simulink model "definitivo"  (R2023a)
settings: Solver=VariableStepAuto  StartTime=0.0  StopTime=T_sim  RelTol=1e-3
values from neighbouring files (symbols this model uses):
  k = 1    [main.m]
  mu = 0.5    [main.m]
undefined symbols (not defined in the file or in its folder): A_tubo, base_barile, c, d_tubo, do_percent, g, gamma_l, h_limite, k_imbocco, k_uscita, kg_to_m, l, L_tubo, livello_0, m_to_kg, mu_l, p1, p2, r, r_grande, r_piccolo, rho_l, step_liq, step_time, theta_grande, theta_piccolo, up_percent, z1, z2
libraries: simulink x8
settings Model: Creator=PaoloA  LastModifiedBy=PaoloA

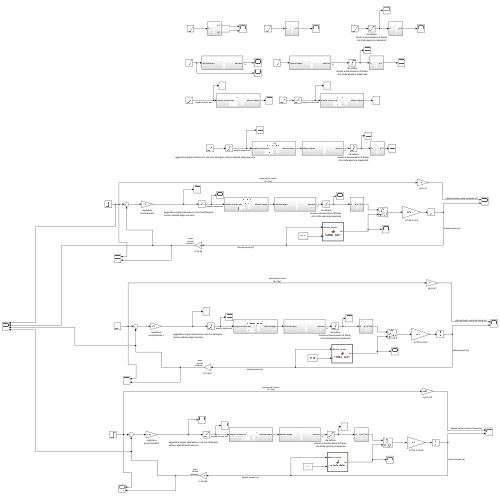
[thumbnail: Simulink's stored preview of the top-level diagram]
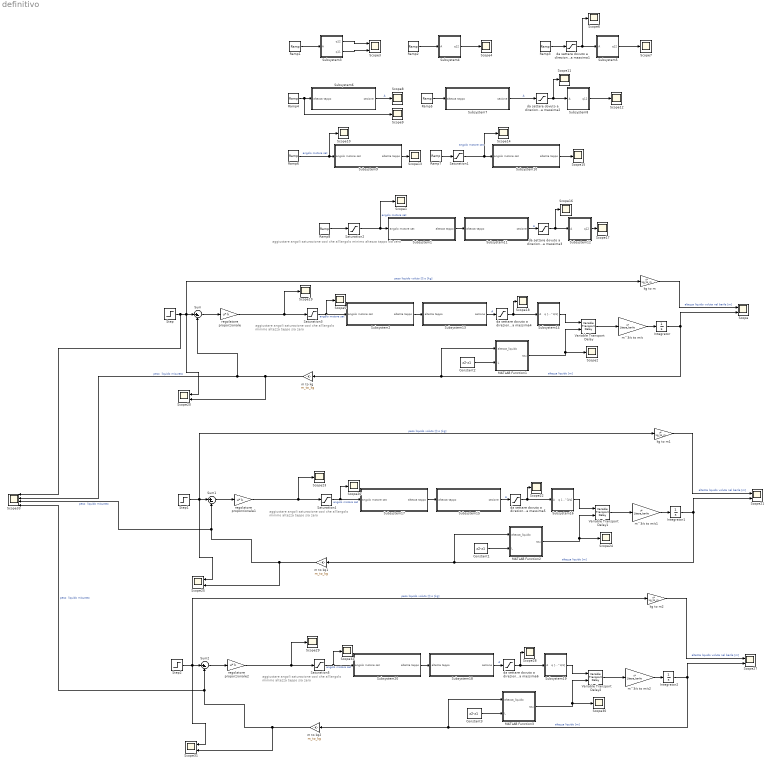
== system definitivo ==
  note: aggiustare angoli saturazione così che all'angolo minimo altezza tappo sia zero
  note: aggiustare angoli saturazione così che all'angolo
      | minimo altezza tappo sia zero
  note: aggiustare angoli saturazione così che all'angolo
      | minimo altezza tappo sia zero
  note: aggiustare angoli saturazione così che all'angolo
      | minimo altezza tappo sia zero
  Constant1 : Constant  Value=z2-z1
  Constant2 : Constant  Value=z2-z1
  Constant3 : Constant  Value=z2-z1
  Integrator : Integrator  InitialCondition=livello_0
  Integrator1 : Integrator  InitialCondition=livello_0
  Integrator2 : Integrator  InitialCondition=livello_0
  MATLAB Function1 : MATLAB Function  TreatAsAtomicUnit=on
  MATLAB Function2 : MATLAB Function  TreatAsAtomicUnit=on
  MATLAB Function3 : MATLAB Function  TreatAsAtomicUnit=on
  Ramp1 : simulink/Sources/Ramp  slope=0.00001  start=5  InitialOutput=0
  Ramp2 : simulink/Sources/Ramp  slope=0.00001  start=5  InitialOutput=0
  Ramp3 : simulink/Sources/Ramp  slope=0.00001  start=5  InitialOutput=0
  Ramp4 : simulink/Sources/Ramp  slope=0.0005  start=5  InitialOutput=0
  Ramp5 : simulink/Sources/Ramp  slope=0.0005  start=5  InitialOutput=0
  Ramp6 : simulink/Sources/Ramp  slope=0.2  start=5  InitialOutput=0
  Ramp7 : simulink/Sources/Ramp  slope=0.03  start=5  InitialOutput=0
  Ramp8 : simulink/Sources/Ramp  slope=0.03  start=5  InitialOutput=0
  Saturation{1..5} (5 alike) : Saturate  UpperLimit=pi  LowerLimit=0.01
  Scope{,3,20..21,25,27,31} (7 alike) : Scope  NumInputPorts=2
  Scope{1..2,4..19,22..24,26,28..30,32} (26 alike) : Scope
  Scope33 : Scope  NumInputPorts=4
  Step : Step  Time=step_time  After=step_liq  SampleTime=0
  Step1 : Step  Time=step_time  After=step_liq  SampleTime=0
  Step2 : Step  Time=step_time  After=step_liq  SampleTime=0
  Subsystem1 : Subsystem
  Subsystem10 : Subsystem
  Subsystem11 : Subsystem
  Subsystem12 : Subsystem
  Subsystem13 : Subsystem
  Subsystem14 : Subsystem
  Subsystem15 : Subsystem
  Subsystem16 : Subsystem
  Subsystem17 : Subsystem
  Subsystem18 : Subsystem
  Subsystem19 : Subsystem
  Subsystem2 : Subsystem
  Subsystem20 : Subsystem
  Subsystem3 : Subsystem
  Subsystem4 : Subsystem
  Subsystem5 : Subsystem
  Subsystem6 : Subsystem
  Subsystem7 : Subsystem
  Subsystem8 : Subsystem
  Subsystem9 : Subsystem
  Sum : Sum  Inputs=|+-
  Sum1 : Sum  Inputs=|+-
  Sum2 : Sum  Inputs=|+-
  Variable Transport Delay : VariableTransportDelay  MaximumDelay=tau_max
  Variable Transport Delay1 : VariableTransportDelay  MaximumDelay=tau_max
  Variable Transport Delay2 : VariableTransportDelay  MaximumDelay=tau_max
  da settare dovuto a direzionatore di flusso che limita apertura massima{1..6} (6 alike) : Saturate  UpperLimit=100  LowerLimit=0
  kg to m : Gain  Gain=kg_to_m  Multiplication=Matrix(u*K)
  kg to m1 : Gain  Gain=kg_to_m  Multiplication=Matrix(u*K)
  kg to m2 : Gain  Gain=kg_to_m  Multiplication=Matrix(u*K)
  m to kg : Gain  Gain=m_to_kg
  m to kg1 : Gain  Gain=m_to_kg
  m to kg2 : Gain  Gain=m_to_kg
  m^3/s to m/s : Gain  Gain=1/base_barile  Multiplication=Matrix(u*K)
  m^3/s to m/s1 : Gain  Gain=1/base_barile  Multiplication=Matrix(u*K)
  m^3/s to m/s2 : Gain  Gain=1/base_barile  Multiplication=Matrix(u*K)
  regolatore proporzionale : Gain  Gain=k  Multiplication=Matrix(u*K)
  regolatore proporzionale1 : Gain  Gain=k  Multiplication=Matrix(u*K)
  regolatore proporzionale2 : Gain  Gain=k  Multiplication=Matrix(u*K)
  wires:
  Subsystem3/1(q12) -> Scope3/1
  Subsystem4/1(q12) -> Scope4/1
  Sum/1 -> regolatore proporzionale/1
  Subsystem11/1(sezione) -> da settare dovuto a direzionatore di flusso che limita apertura massima3/1  "A"
  Step/1 -> Scope33/1, Scope20/1, kg to m/1, Sum/1  "peso liquido voluto [l] o [kg]"
  Ramp6/1 -> Scope10/1, Subsystem9/1(angolo motore sat)  "angolo motore sat"
  Subsystem12/1(q12) -> Scope17/1
  Integrator/1 -> m to kg/1, MATLAB Function1/1(altezza_liquido), Scope/2  "altezza liquido [m]"
  Subsystem9/1(altezza tappo) -> Scope13/1
  Saturation3/1 -> Subsystem2/1(angolo motore sat), Scope5/1  "angolo motore sat"
  regolatore proporzionale/1 -> Scope19/1, Saturation3/1
  Subsystem2/1(altezza tappo) -> Subsystem13/1(altezza tappo)
  MATLAB Function1/1(tau) -> Variable Transport Delay/2, Scope2/1
  da settare dovuto a direzionatore di flusso che limita apertura massima4/1 -> Scope18/1, Subsystem14/1(A)
  m to kg/1 -> Scope33/2, Sum/2, Scope20/2  "peso  liquido misurato"
  m^3/s to m/s/1 -> Integrator/1
  Ramp2/1 -> Subsystem4/1(A)
  Constant2/1 -> MATLAB Function1/2(L)
  Ramp7/1 -> Saturation1/1
  Subsystem8/1(q12) -> Scope12/1
  Saturation2/1 -> Scope1/1, Subsystem1/1(angolo motore sat)  "angolo motore sat"
  Subsystem1/1(altezza tappo) -> Subsystem11/1(altezza tappo)
  Ramp5/1 -> Subsystem7/1(altezza tappo)
  Subsystem13/1(sezione) -> da settare dovuto a direzionatore di flusso che limita apertura massima4/1  "A"
  Subsystem10/1(altezza tappo) -> Scope15/1
  Saturation1/1 -> Scope14/1, Subsystem10/1(angolo motore sat)  "angolo motore sat"
  da settare dovuto a direzionatore di flusso che limita apertura massima2/1 -> Scope11/1, Subsystem8/1(A)
  Variable Transport Delay/1 -> m^3/s to m/s/1
  Ramp4/1 -> Scope9/1, Subsystem6/1(altezza tappo)
  Ramp8/1 -> Saturation2/1
  Subsystem6/1(sezione) -> Scope8/1  "A"
  Ramp3/1 -> da settare dovuto a direzionatore di flusso che limita apertura massima1/1
  da settare dovuto a direzionatore di flusso che limita apertura massima1/1 -> Scope6/1, Subsystem5/1(A)
  Subsystem3/2(q11) -> Scope3/2
  Subsystem7/1(sezione) -> da settare dovuto a direzionatore di flusso che limita apertura massima2/1  "A"
  da settare dovuto a direzionatore di flusso che limita apertura massima3/1 -> Scope16/1, Subsystem12/1(A)
  Subsystem14/1(q [m^3/s]) -> Variable Transport Delay/1
  Ramp1/1 -> Subsystem3/1(A)
  Subsystem5/1(q12) -> Scope7/1
  kg to m/1 -> Scope/1  "altezza liquido voluta nel barile [m]"
  Step1/1 -> Scope25/1, kg to m1/1, Sum1/1  "peso liquido voluto [l] o [kg]"
  Integrator1/1 -> m to kg1/1, MATLAB Function2/1(altezza_liquido), Scope21/2  "altezza liquido [m]"
  da settare dovuto a direzionatore di flusso che limita apertura massima5/1 -> Scope22/1, Subsystem16/1(A)
  m^3/s to m/s1/1 -> Integrator1/1
  regolatore proporzionale1/1 -> Scope23/1, Saturation4/1
  Subsystem17/1(altezza tappo) -> Subsystem15/1(altezza tappo)
  Sum1/1 -> regolatore proporzionale1/1
  Saturation4/1 -> Subsystem17/1(angolo motore sat), Scope26/1  "angolo motore sat"
  Constant1/1 -> MATLAB Function2/2(L)
  kg to m1/1 -> Scope21/1  "altezza liquido voluta nel barile [m]"
  MATLAB Function2/1(tau) -> Variable Transport Delay1/2, Scope24/1
  Subsystem16/1(q [m^3/s]) -> Variable Transport Delay1/1
  m to kg1/1 -> Scope33/3, Sum1/2, Scope25/2  "peso  liquido misurato"
  Subsystem15/1(sezione) -> da settare dovuto a direzionatore di flusso che limita apertura massima5/1  "A"
  Variable Transport Delay1/1 -> m^3/s to m/s1/1
  Variable Transport Delay2/1 -> m^3/s to m/s2/1
  Subsystem18/1(sezione) -> da settare dovuto a direzionatore di flusso che limita apertura massima6/1  "A"
  MATLAB Function3/1(tau) -> Variable Transport Delay2/2, Scope30/1
  kg to m2/1 -> Scope27/1  "altezza liquido voluta nel barile [m]"
  Subsystem20/1(altezza tappo) -> Subsystem18/1(altezza tappo)
  Subsystem19/1(q [m^3/s]) -> Variable Transport Delay2/1
  Integrator2/1 -> m to kg2/1, MATLAB Function3/1(altezza_liquido), Scope27/2  "altezza liquido [m]"
  Constant3/1 -> MATLAB Function3/2(L)
  m^3/s to m/s2/1 -> Integrator2/1
  da settare dovuto a direzionatore di flusso che limita apertura massima6/1 -> Scope28/1, Subsystem19/1(A)
  m to kg2/1 -> Scope33/4, Sum2/2, Scope31/2  "peso  liquido misurato"
  Saturation5/1 -> Subsystem20/1(angolo motore sat), Scope32/1  "angolo motore sat"
  regolatore proporzionale2/1 -> Scope29/1, Saturation5/1
  Step2/1 -> Scope31/1, kg to m2/1, Sum2/1  "peso liquido voluto [l] o [kg]"
  Sum2/1 -> regolatore proporzionale2/1

== system definitivo/Subsystem1 ==
  note: sistemare
  angolo motore sat : Inport
  Constant : Constant  Value=r
  Constant1 : Constant  Value=l
  Constant2 : Constant  Value=mu
  MATLAB Function : MATLAB Function  TreatAsAtomicUnit=on
  altezza tappo : Outport
  wires:
  Constant/1 -> MATLAB Function/2(r)
  MATLAB Function/1(h_tappo) -> altezza tappo/1  "altezza tappo"
  angolo motore sat/1 -> MATLAB Function/1(alpha)
  Constant1/1 -> MATLAB Function/3(l)
  Constant2/1 -> MATLAB Function/4(mu)

== system definitivo/Subsystem10 ==
  note: sistemare
  angolo motore sat : Inport
  Constant : Constant  Value=r
  Constant1 : Constant  Value=l
  Constant2 : Constant  Value=mu
  MATLAB Function : MATLAB Function  TreatAsAtomicUnit=on
  altezza tappo : Outport
  wires:
  Constant/1 -> MATLAB Function/2(r)
  MATLAB Function/1(h_tappo) -> altezza tappo/1  "altezza tappo"
  angolo motore sat/1 -> MATLAB Function/1(alpha)
  Constant1/1 -> MATLAB Function/3(l)
  Constant2/1 -> MATLAB Function/4(mu)

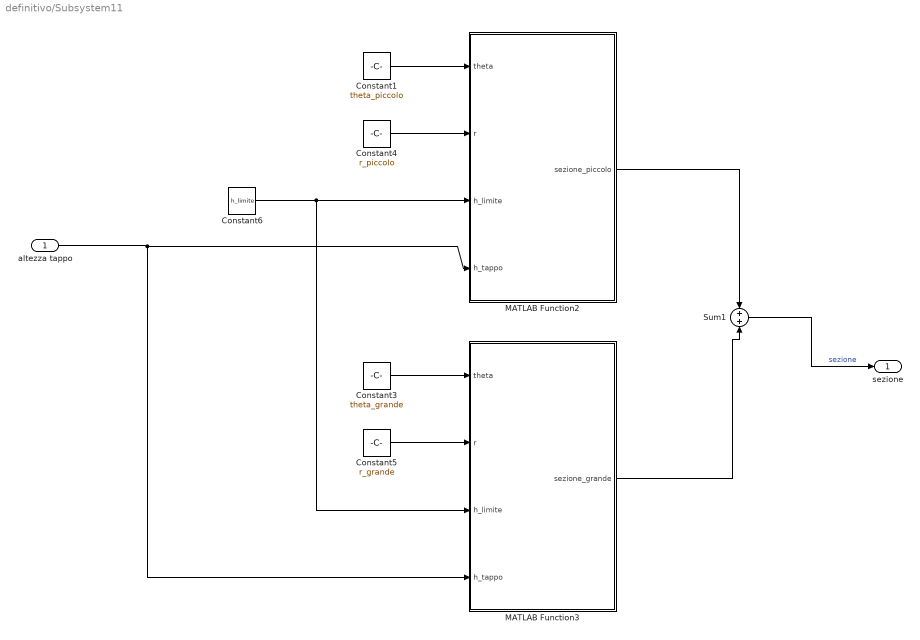
== system definitivo/Subsystem11 ==
  altezza tappo : Inport
  Constant1 : Constant  Value=theta_piccolo
  Constant3 : Constant  Value=theta_grande  VectorParams1D=off
  Constant4 : Constant  Value=r_piccolo
  Constant5 : Constant  Value=r_grande
  Constant6 : Constant  Value=h_limite
  MATLAB Function2 : MATLAB Function  TreatAsAtomicUnit=on
  MATLAB Function3 : MATLAB Function  TreatAsAtomicUnit=on
  Sum1 : Sum
  sezione : Outport
  wires:
  MATLAB Function2/1(sezione_piccolo) -> Sum1/1
  altezza tappo/1 -> MATLAB Function3/4(h_tappo), MATLAB Function2/4(h_tappo)
  Constant3/1 -> MATLAB Function3/1(theta)
  Constant5/1 -> MATLAB Function3/2(r)
  Constant4/1 -> MATLAB Function2/2(r)
  Sum1/1 -> sezione/1  "sezione"
  MATLAB Function3/1(sezione_grande) -> Sum1/2
  Constant1/1 -> MATLAB Function2/1(theta)
  Constant6/1 -> MATLAB Function3/3(h_limite), MATLAB Function2/3(h_limite)

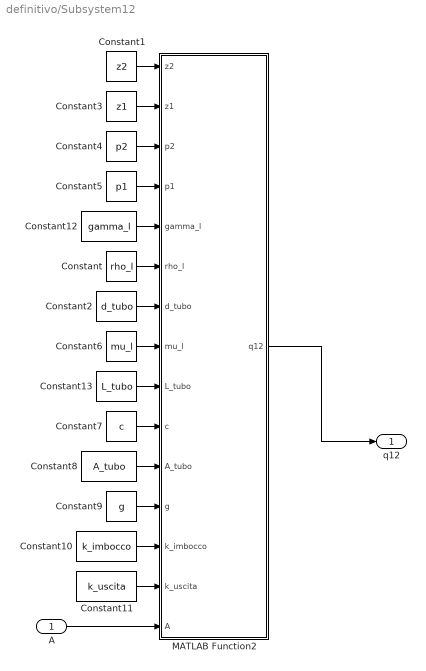
== system definitivo/Subsystem12 ==
  A : Inport
  Constant : Constant  Value=rho_l
  Constant1 : Constant  Value=z2
  Constant10 : Constant  Value=k_imbocco
  Constant11 : Constant  Value=k_uscita
  Constant12 : Constant  Value=gamma_l
  Constant13 : Constant  Value=L_tubo
  Constant2 : Constant  Value=d_tubo
  Constant3 : Constant  Value=z1
  Constant4 : Constant  Value=p2
  Constant5 : Constant  Value=p1
  Constant6 : Constant  Value=mu_l
  Constant7 : Constant  Value=c
  Constant8 : Constant  Value=A_tubo
  Constant9 : Constant  Value=g
  MATLAB Function2 : MATLAB Function  TreatAsAtomicUnit=on
  q12 : Outport
  wires:
  Constant11/1 -> MATLAB Function2/14(k_uscita)
  Constant5/1 -> MATLAB Function2/4(p1)
  Constant3/1 -> MATLAB Function2/2(z1)
  Constant10/1 -> MATLAB Function2/13(k_imbocco)
  Constant9/1 -> MATLAB Function2/12(g)
  Constant/1 -> MATLAB Function2/6(rho_l)
  Constant1/1 -> MATLAB Function2/1(z2)
  Constant4/1 -> MATLAB Function2/3(p2)
  Constant7/1 -> MATLAB Function2/10(c)
  Constant12/1 -> MATLAB Function2/5(gamma_l)
  Constant8/1 -> MATLAB Function2/11(A_tubo)
  A/1 -> MATLAB Function2/15(A)
  Constant2/1 -> MATLAB Function2/7(d_tubo)
  Constant6/1 -> MATLAB Function2/8(mu_l)
  Constant13/1 -> MATLAB Function2/9(L_tubo)
  MATLAB Function2/1(q12) -> q12/1

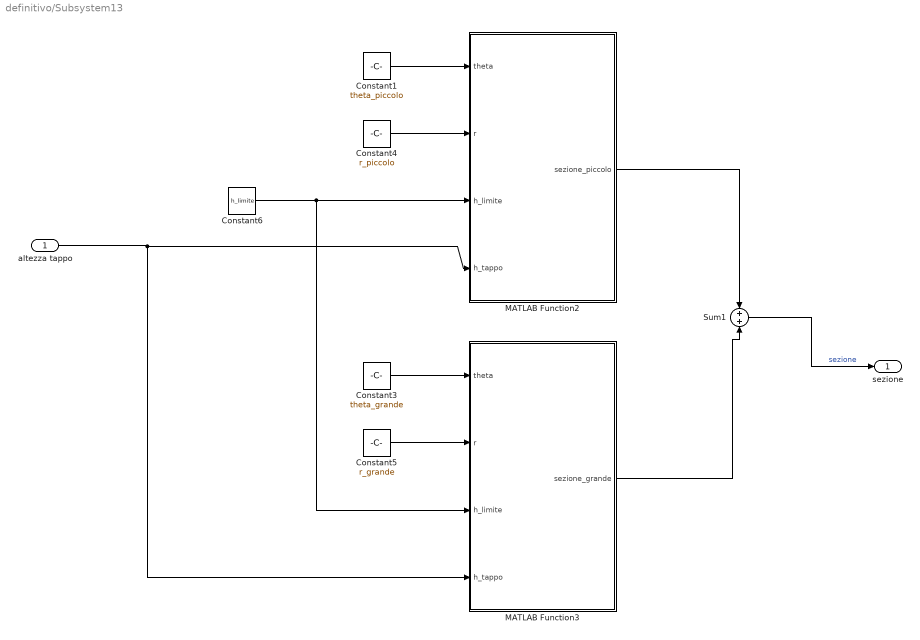
== system definitivo/Subsystem13 ==
  altezza tappo : Inport
  Constant1 : Constant  Value=theta_piccolo
  Constant3 : Constant  Value=theta_grande  VectorParams1D=off
  Constant4 : Constant  Value=r_piccolo
  Constant5 : Constant  Value=r_grande
  Constant6 : Constant  Value=h_limite
  MATLAB Function2 : MATLAB Function  TreatAsAtomicUnit=on
  MATLAB Function3 : MATLAB Function  TreatAsAtomicUnit=on
  Sum1 : Sum
  sezione : Outport
  wires:
  MATLAB Function2/1(sezione_piccolo) -> Sum1/1
  altezza tappo/1 -> MATLAB Function3/4(h_tappo), MATLAB Function2/4(h_tappo)
  Constant3/1 -> MATLAB Function3/1(theta)
  Constant5/1 -> MATLAB Function3/2(r)
  Constant4/1 -> MATLAB Function2/2(r)
  Sum1/1 -> sezione/1  "sezione"
  MATLAB Function3/1(sezione_grande) -> Sum1/2
  Constant1/1 -> MATLAB Function2/1(theta)
  Constant6/1 -> MATLAB Function3/3(h_limite), MATLAB Function2/3(h_limite)

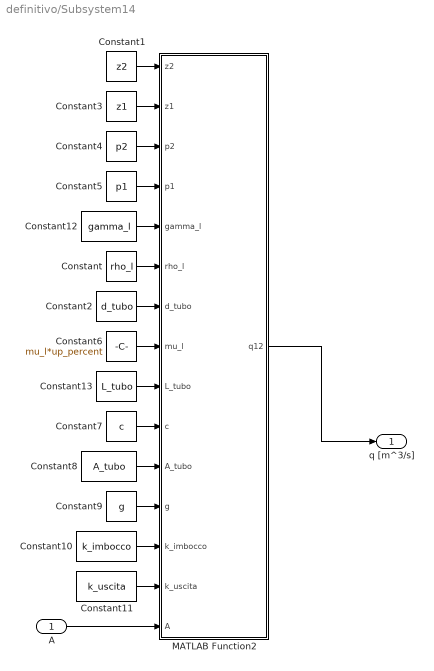
== system definitivo/Subsystem14 ==
  A : Inport
  Constant : Constant  Value=rho_l
  Constant1 : Constant  Value=z2
  Constant10 : Constant  Value=k_imbocco
  Constant11 : Constant  Value=k_uscita
  Constant12 : Constant  Value=gamma_l
  Constant13 : Constant  Value=L_tubo
  Constant2 : Constant  Value=d_tubo
  Constant3 : Constant  Value=z1
  Constant4 : Constant  Value=p2
  Constant5 : Constant  Value=p1
  Constant6 : Constant  Value=mu_l*up_percent
  Constant7 : Constant  Value=c
  Constant8 : Constant  Value=A_tubo
  Constant9 : Constant  Value=g
  MATLAB Function2 : MATLAB Function  TreatAsAtomicUnit=on
  q [m^3/s] : Outport
  wires:
  Constant11/1 -> MATLAB Function2/14(k_uscita)
  Constant5/1 -> MATLAB Function2/4(p1)
  Constant3/1 -> MATLAB Function2/2(z1)
  Constant10/1 -> MATLAB Function2/13(k_imbocco)
  Constant9/1 -> MATLAB Function2/12(g)
  Constant/1 -> MATLAB Function2/6(rho_l)
  Constant1/1 -> MATLAB Function2/1(z2)
  Constant4/1 -> MATLAB Function2/3(p2)
  Constant7/1 -> MATLAB Function2/10(c)
  Constant12/1 -> MATLAB Function2/5(gamma_l)
  Constant8/1 -> MATLAB Function2/11(A_tubo)
  A/1 -> MATLAB Function2/15(A)
  Constant2/1 -> MATLAB Function2/7(d_tubo)
  Constant6/1 -> MATLAB Function2/8(mu_l)
  Constant13/1 -> MATLAB Function2/9(L_tubo)
  MATLAB Function2/1(q12) -> q [m^3/s]/1

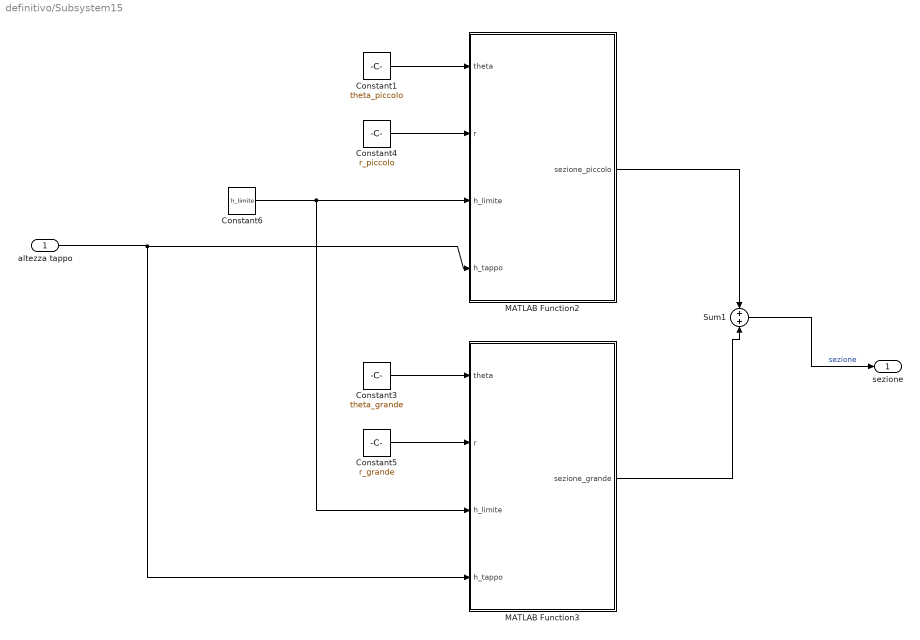
== system definitivo/Subsystem15 ==
  altezza tappo : Inport
  Constant1 : Constant  Value=theta_piccolo
  Constant3 : Constant  Value=theta_grande  VectorParams1D=off
  Constant4 : Constant  Value=r_piccolo
  Constant5 : Constant  Value=r_grande
  Constant6 : Constant  Value=h_limite
  MATLAB Function2 : MATLAB Function  TreatAsAtomicUnit=on
  MATLAB Function3 : MATLAB Function  TreatAsAtomicUnit=on
  Sum1 : Sum
  sezione : Outport
  wires:
  MATLAB Function2/1(sezione_piccolo) -> Sum1/1
  altezza tappo/1 -> MATLAB Function3/4(h_tappo), MATLAB Function2/4(h_tappo)
  Constant3/1 -> MATLAB Function3/1(theta)
  Constant5/1 -> MATLAB Function3/2(r)
  Constant4/1 -> MATLAB Function2/2(r)
  Sum1/1 -> sezione/1  "sezione"
  MATLAB Function3/1(sezione_grande) -> Sum1/2
  Constant1/1 -> MATLAB Function2/1(theta)
  Constant6/1 -> MATLAB Function3/3(h_limite), MATLAB Function2/3(h_limite)

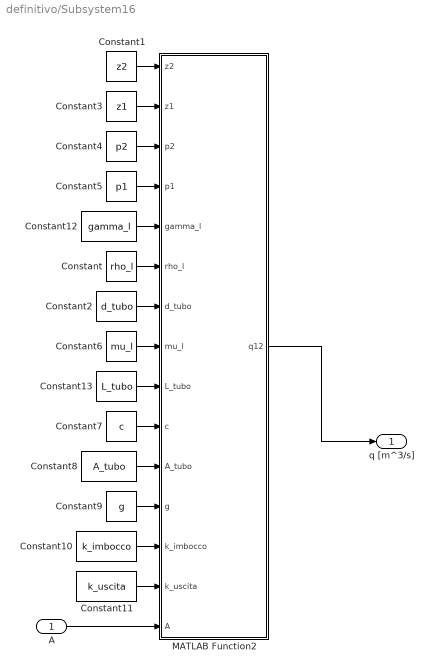
== system definitivo/Subsystem16 ==
  A : Inport
  Constant : Constant  Value=rho_l
  Constant1 : Constant  Value=z2
  Constant10 : Constant  Value=k_imbocco
  Constant11 : Constant  Value=k_uscita
  Constant12 : Constant  Value=gamma_l
  Constant13 : Constant  Value=L_tubo
  Constant2 : Constant  Value=d_tubo
  Constant3 : Constant  Value=z1
  Constant4 : Constant  Value=p2
  Constant5 : Constant  Value=p1
  Constant6 : Constant  Value=mu_l
  Constant7 : Constant  Value=c
  Constant8 : Constant  Value=A_tubo
  Constant9 : Constant  Value=g
  MATLAB Function2 : MATLAB Function  TreatAsAtomicUnit=on
  q [m^3/s] : Outport
  wires:
  Constant11/1 -> MATLAB Function2/14(k_uscita)
  Constant5/1 -> MATLAB Function2/4(p1)
  Constant3/1 -> MATLAB Function2/2(z1)
  Constant10/1 -> MATLAB Function2/13(k_imbocco)
  Constant9/1 -> MATLAB Function2/12(g)
  Constant/1 -> MATLAB Function2/6(rho_l)
  Constant1/1 -> MATLAB Function2/1(z2)
  Constant4/1 -> MATLAB Function2/3(p2)
  Constant7/1 -> MATLAB Function2/10(c)
  Constant12/1 -> MATLAB Function2/5(gamma_l)
  Constant8/1 -> MATLAB Function2/11(A_tubo)
  A/1 -> MATLAB Function2/15(A)
  Constant2/1 -> MATLAB Function2/7(d_tubo)
  Constant6/1 -> MATLAB Function2/8(mu_l)
  Constant13/1 -> MATLAB Function2/9(L_tubo)
  MATLAB Function2/1(q12) -> q [m^3/s]/1

== system definitivo/Subsystem17 ==
  note: sistemare
  angolo motore sat : Inport
  Constant : Constant  Value=r
  Constant1 : Constant  Value=l
  Constant2 : Constant  Value=mu
  MATLAB Function : MATLAB Function  TreatAsAtomicUnit=on
  altezza tappo : Outport
  wires:
  Constant/1 -> MATLAB Function/2(r)
  MATLAB Function/1(h_tappo) -> altezza tappo/1  "altezza tappo"
  angolo motore sat/1 -> MATLAB Function/1(alpha)
  Constant1/1 -> MATLAB Function/3(l)
  Constant2/1 -> MATLAB Function/4(mu)

== system definitivo/Subsystem18 ==
  altezza tappo : Inport
  Constant1 : Constant  Value=theta_piccolo
  Constant3 : Constant  Value=theta_grande  VectorParams1D=off
  Constant4 : Constant  Value=r_piccolo
  Constant5 : Constant  Value=r_grande
  Constant6 : Constant  Value=h_limite
  MATLAB Function2 : MATLAB Function  TreatAsAtomicUnit=on
  MATLAB Function3 : MATLAB Function  TreatAsAtomicUnit=on
  Sum1 : Sum
  sezione : Outport
  wires:
  MATLAB Function2/1(sezione_piccolo) -> Sum1/1
  altezza tappo/1 -> MATLAB Function3/4(h_tappo), MATLAB Function2/4(h_tappo)
  Constant3/1 -> MATLAB Function3/1(theta)
  Constant5/1 -> MATLAB Function3/2(r)
  Constant4/1 -> MATLAB Function2/2(r)
  Sum1/1 -> sezione/1  "sezione"
  MATLAB Function3/1(sezione_grande) -> Sum1/2
  Constant1/1 -> MATLAB Function2/1(theta)
  Constant6/1 -> MATLAB Function3/3(h_limite), MATLAB Function2/3(h_limite)

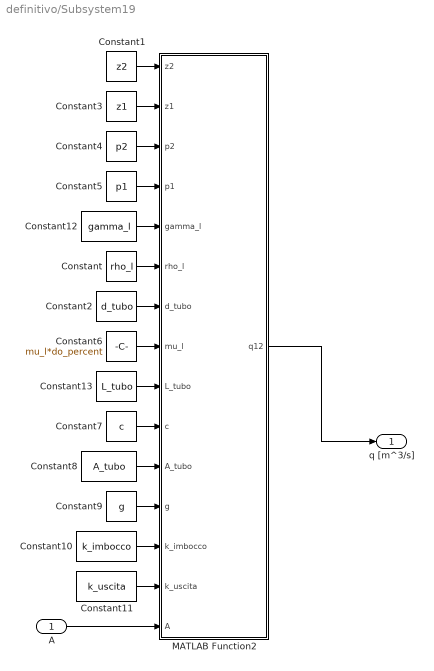
== system definitivo/Subsystem19 ==
  A : Inport
  Constant : Constant  Value=rho_l
  Constant1 : Constant  Value=z2
  Constant10 : Constant  Value=k_imbocco
  Constant11 : Constant  Value=k_uscita
  Constant12 : Constant  Value=gamma_l
  Constant13 : Constant  Value=L_tubo
  Constant2 : Constant  Value=d_tubo
  Constant3 : Constant  Value=z1
  Constant4 : Constant  Value=p2
  Constant5 : Constant  Value=p1
  Constant6 : Constant  Value=mu_l*do_percent
  Constant7 : Constant  Value=c
  Constant8 : Constant  Value=A_tubo
  Constant9 : Constant  Value=g
  MATLAB Function2 : MATLAB Function  TreatAsAtomicUnit=on
  q [m^3/s] : Outport
  wires:
  Constant11/1 -> MATLAB Function2/14(k_uscita)
  Constant5/1 -> MATLAB Function2/4(p1)
  Constant3/1 -> MATLAB Function2/2(z1)
  Constant10/1 -> MATLAB Function2/13(k_imbocco)
  Constant9/1 -> MATLAB Function2/12(g)
  Constant/1 -> MATLAB Function2/6(rho_l)
  Constant1/1 -> MATLAB Function2/1(z2)
  Constant4/1 -> MATLAB Function2/3(p2)
  Constant7/1 -> MATLAB Function2/10(c)
  Constant12/1 -> MATLAB Function2/5(gamma_l)
  Constant8/1 -> MATLAB Function2/11(A_tubo)
  A/1 -> MATLAB Function2/15(A)
  Constant2/1 -> MATLAB Function2/7(d_tubo)
  Constant6/1 -> MATLAB Function2/8(mu_l)
  Constant13/1 -> MATLAB Function2/9(L_tubo)
  MATLAB Function2/1(q12) -> q [m^3/s]/1

== system definitivo/Subsystem2 ==
  note: sistemare
  angolo motore sat : Inport
  Constant : Constant  Value=r
  Constant1 : Constant  Value=l
  Constant2 : Constant  Value=mu
  MATLAB Function : MATLAB Function  TreatAsAtomicUnit=on
  altezza tappo : Outport
  wires:
  Constant/1 -> MATLAB Function/2(r)
  MATLAB Function/1(h_tappo) -> altezza tappo/1  "altezza tappo"
  angolo motore sat/1 -> MATLAB Function/1(alpha)
  Constant1/1 -> MATLAB Function/3(l)
  Constant2/1 -> MATLAB Function/4(mu)

== system definitivo/Subsystem20 ==
  note: sistemare
  angolo motore sat : Inport
  Constant : Constant  Value=r
  Constant1 : Constant  Value=l
  Constant2 : Constant  Value=mu
  MATLAB Function : MATLAB Function  TreatAsAtomicUnit=on
  altezza tappo : Outport
  wires:
  Constant/1 -> MATLAB Function/2(r)
  MATLAB Function/1(h_tappo) -> altezza tappo/1  "altezza tappo"
  angolo motore sat/1 -> MATLAB Function/1(alpha)
  Constant1/1 -> MATLAB Function/3(l)
  Constant2/1 -> MATLAB Function/4(mu)

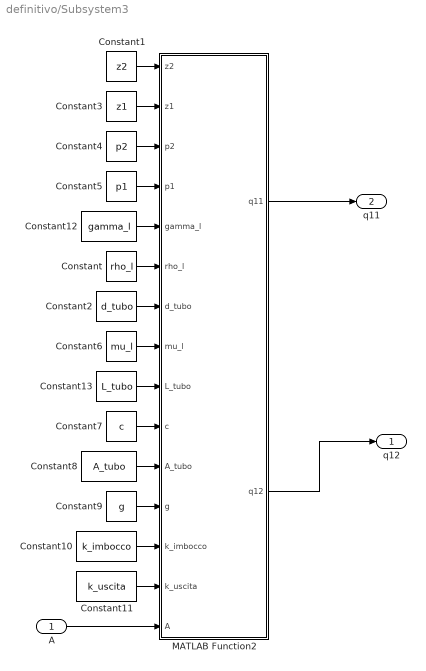
== system definitivo/Subsystem3 ==
  A : Inport
  Constant : Constant  Value=rho_l
  Constant1 : Constant  Value=z2
  Constant10 : Constant  Value=k_imbocco
  Constant11 : Constant  Value=k_uscita
  Constant12 : Constant  Value=gamma_l
  Constant13 : Constant  Value=L_tubo
  Constant2 : Constant  Value=d_tubo
  Constant3 : Constant  Value=z1
  Constant4 : Constant  Value=p2
  Constant5 : Constant  Value=p1
  Constant6 : Constant  Value=mu_l
  Constant7 : Constant  Value=c
  Constant8 : Constant  Value=A_tubo
  Constant9 : Constant  Value=g
  MATLAB Function2 : MATLAB Function  TreatAsAtomicUnit=on
  q12 : Outport
  q11 : Outport  Port=2
  wires:
  Constant11/1 -> MATLAB Function2/14(k_uscita)
  Constant5/1 -> MATLAB Function2/4(p1)
  Constant3/1 -> MATLAB Function2/2(z1)
  Constant10/1 -> MATLAB Function2/13(k_imbocco)
  Constant9/1 -> MATLAB Function2/12(g)
  Constant/1 -> MATLAB Function2/6(rho_l)
  Constant1/1 -> MATLAB Function2/1(z2)
  Constant4/1 -> MATLAB Function2/3(p2)
  Constant7/1 -> MATLAB Function2/10(c)
  Constant12/1 -> MATLAB Function2/5(gamma_l)
  Constant8/1 -> MATLAB Function2/11(A_tubo)
  A/1 -> MATLAB Function2/15(A)
  Constant2/1 -> MATLAB Function2/7(d_tubo)
  Constant6/1 -> MATLAB Function2/8(mu_l)
  Constant13/1 -> MATLAB Function2/9(L_tubo)
  MATLAB Function2/2(q12) -> q12/1
  MATLAB Function2/1(q11) -> q11/1

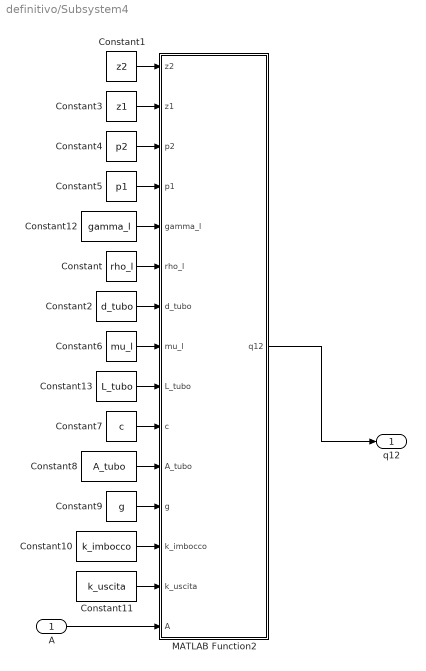
== system definitivo/Subsystem4 ==
  A : Inport
  Constant : Constant  Value=rho_l
  Constant1 : Constant  Value=z2
  Constant10 : Constant  Value=k_imbocco
  Constant11 : Constant  Value=k_uscita
  Constant12 : Constant  Value=gamma_l
  Constant13 : Constant  Value=L_tubo
  Constant2 : Constant  Value=d_tubo
  Constant3 : Constant  Value=z1
  Constant4 : Constant  Value=p2
  Constant5 : Constant  Value=p1
  Constant6 : Constant  Value=mu_l
  Constant7 : Constant  Value=c
  Constant8 : Constant  Value=A_tubo
  Constant9 : Constant  Value=g
  MATLAB Function2 : MATLAB Function  TreatAsAtomicUnit=on
  q12 : Outport
  wires:
  Constant11/1 -> MATLAB Function2/14(k_uscita)
  Constant5/1 -> MATLAB Function2/4(p1)
  Constant3/1 -> MATLAB Function2/2(z1)
  Constant10/1 -> MATLAB Function2/13(k_imbocco)
  Constant9/1 -> MATLAB Function2/12(g)
  Constant/1 -> MATLAB Function2/6(rho_l)
  Constant1/1 -> MATLAB Function2/1(z2)
  Constant4/1 -> MATLAB Function2/3(p2)
  Constant7/1 -> MATLAB Function2/10(c)
  Constant12/1 -> MATLAB Function2/5(gamma_l)
  Constant8/1 -> MATLAB Function2/11(A_tubo)
  A/1 -> MATLAB Function2/15(A)
  Constant2/1 -> MATLAB Function2/7(d_tubo)
  Constant6/1 -> MATLAB Function2/8(mu_l)
  Constant13/1 -> MATLAB Function2/9(L_tubo)
  MATLAB Function2/1(q12) -> q12/1

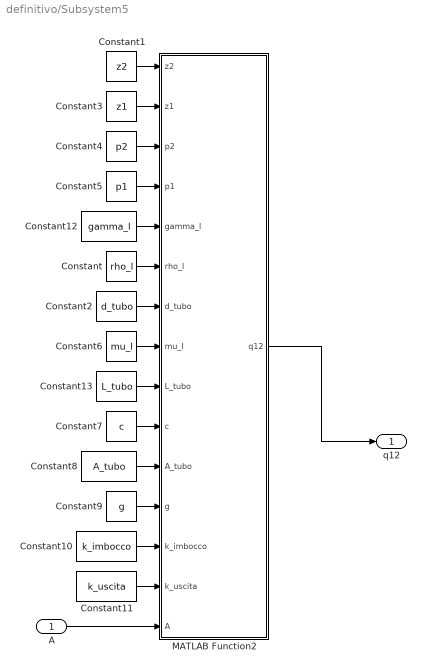
== system definitivo/Subsystem5 ==
  A : Inport
  Constant : Constant  Value=rho_l
  Constant1 : Constant  Value=z2
  Constant10 : Constant  Value=k_imbocco
  Constant11 : Constant  Value=k_uscita
  Constant12 : Constant  Value=gamma_l
  Constant13 : Constant  Value=L_tubo
  Constant2 : Constant  Value=d_tubo
  Constant3 : Constant  Value=z1
  Constant4 : Constant  Value=p2
  Constant5 : Constant  Value=p1
  Constant6 : Constant  Value=mu_l
  Constant7 : Constant  Value=c
  Constant8 : Constant  Value=A_tubo
  Constant9 : Constant  Value=g
  MATLAB Function2 : MATLAB Function  TreatAsAtomicUnit=on
  q12 : Outport
  wires:
  Constant11/1 -> MATLAB Function2/14(k_uscita)
  Constant5/1 -> MATLAB Function2/4(p1)
  Constant3/1 -> MATLAB Function2/2(z1)
  Constant10/1 -> MATLAB Function2/13(k_imbocco)
  Constant9/1 -> MATLAB Function2/12(g)
  Constant/1 -> MATLAB Function2/6(rho_l)
  Constant1/1 -> MATLAB Function2/1(z2)
  Constant4/1 -> MATLAB Function2/3(p2)
  Constant7/1 -> MATLAB Function2/10(c)
  Constant12/1 -> MATLAB Function2/5(gamma_l)
  Constant8/1 -> MATLAB Function2/11(A_tubo)
  A/1 -> MATLAB Function2/15(A)
  Constant2/1 -> MATLAB Function2/7(d_tubo)
  Constant6/1 -> MATLAB Function2/8(mu_l)
  Constant13/1 -> MATLAB Function2/9(L_tubo)
  MATLAB Function2/1(q12) -> q12/1

== system definitivo/Subsystem6 ==
  altezza tappo : Inport
  Constant1 : Constant  Value=theta_piccolo
  Constant3 : Constant  Value=theta_grande  VectorParams1D=off
  Constant4 : Constant  Value=r_piccolo
  Constant5 : Constant  Value=r_grande
  Constant6 : Constant  Value=h_limite
  MATLAB Function2 : MATLAB Function  TreatAsAtomicUnit=on
  MATLAB Function3 : MATLAB Function  TreatAsAtomicUnit=on
  Sum1 : Sum
  sezione : Outport
  wires:
  MATLAB Function2/1(sezione_piccolo) -> Sum1/1
  altezza tappo/1 -> MATLAB Function3/4(h_tappo), MATLAB Function2/4(h_tappo)
  Constant3/1 -> MATLAB Function3/1(theta)
  Constant5/1 -> MATLAB Function3/2(r)
  Constant4/1 -> MATLAB Function2/2(r)
  Sum1/1 -> sezione/1  "sezione"
  MATLAB Function3/1(sezione_grande) -> Sum1/2
  Constant1/1 -> MATLAB Function2/1(theta)
  Constant6/1 -> MATLAB Function3/3(h_limite), MATLAB Function2/3(h_limite)

== system definitivo/Subsystem7 ==
  altezza tappo : Inport
  Constant1 : Constant  Value=theta_piccolo
  Constant3 : Constant  Value=theta_grande  VectorParams1D=off
  Constant4 : Constant  Value=r_piccolo
  Constant5 : Constant  Value=r_grande
  Constant6 : Constant  Value=h_limite
  MATLAB Function2 : MATLAB Function  TreatAsAtomicUnit=on
  MATLAB Function3 : MATLAB Function  TreatAsAtomicUnit=on
  Sum1 : Sum
  sezione : Outport
  wires:
  MATLAB Function2/1(sezione_piccolo) -> Sum1/1
  altezza tappo/1 -> MATLAB Function3/4(h_tappo), MATLAB Function2/4(h_tappo)
  Constant3/1 -> MATLAB Function3/1(theta)
  Constant5/1 -> MATLAB Function3/2(r)
  Constant4/1 -> MATLAB Function2/2(r)
  Sum1/1 -> sezione/1  "sezione"
  MATLAB Function3/1(sezione_grande) -> Sum1/2
  Constant1/1 -> MATLAB Function2/1(theta)
  Constant6/1 -> MATLAB Function3/3(h_limite), MATLAB Function2/3(h_limite)

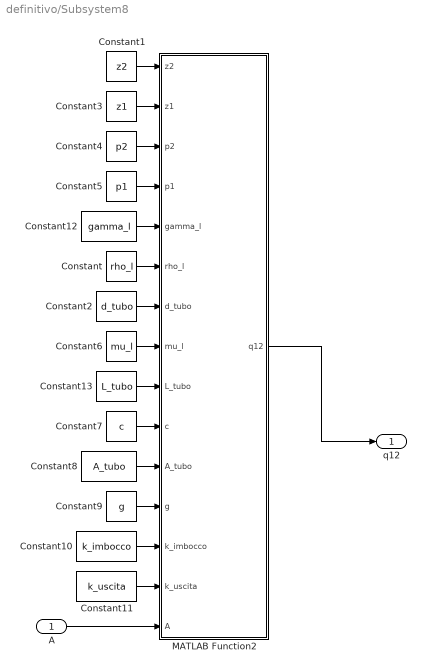
== system definitivo/Subsystem8 ==
  A : Inport
  Constant : Constant  Value=rho_l
  Constant1 : Constant  Value=z2
  Constant10 : Constant  Value=k_imbocco
  Constant11 : Constant  Value=k_uscita
  Constant12 : Constant  Value=gamma_l
  Constant13 : Constant  Value=L_tubo
  Constant2 : Constant  Value=d_tubo
  Constant3 : Constant  Value=z1
  Constant4 : Constant  Value=p2
  Constant5 : Constant  Value=p1
  Constant6 : Constant  Value=mu_l
  Constant7 : Constant  Value=c
  Constant8 : Constant  Value=A_tubo
  Constant9 : Constant  Value=g
  MATLAB Function2 : MATLAB Function  TreatAsAtomicUnit=on
  q12 : Outport
  wires:
  Constant11/1 -> MATLAB Function2/14(k_uscita)
  Constant5/1 -> MATLAB Function2/4(p1)
  Constant3/1 -> MATLAB Function2/2(z1)
  Constant10/1 -> MATLAB Function2/13(k_imbocco)
  Constant9/1 -> MATLAB Function2/12(g)
  Constant/1 -> MATLAB Function2/6(rho_l)
  Constant1/1 -> MATLAB Function2/1(z2)
  Constant4/1 -> MATLAB Function2/3(p2)
  Constant7/1 -> MATLAB Function2/10(c)
  Constant12/1 -> MATLAB Function2/5(gamma_l)
  Constant8/1 -> MATLAB Function2/11(A_tubo)
  A/1 -> MATLAB Function2/15(A)
  Constant2/1 -> MATLAB Function2/7(d_tubo)
  Constant6/1 -> MATLAB Function2/8(mu_l)
  Constant13/1 -> MATLAB Function2/9(L_tubo)
  MATLAB Function2/1(q12) -> q12/1

== system definitivo/Subsystem9 ==
  note: sistemare
  angolo motore sat : Inport
  Constant : Constant  Value=r
  Constant1 : Constant  Value=l
  Constant2 : Constant  Value=mu
  MATLAB Function : MATLAB Function  TreatAsAtomicUnit=on
  altezza tappo : Outport
  wires:
  Constant/1 -> MATLAB Function/2(r)
  MATLAB Function/1(h_tappo) -> altezza tappo/1  "altezza tappo"
  angolo motore sat/1 -> MATLAB Function/1(alpha)
  Constant1/1 -> MATLAB Function/3(l)
  Constant2/1 -> MATLAB Function/4(mu)

== matlab function definitivo/Subsystem5/MATLAB Function2 ==
  data: z2 input; z1 input; p2 input; p1 input; gamma_l input; rho_l input; d_tubo input; mu_l input; L_tubo input; c input; A_tubo input; g input; k_imbocco input; k_uscita input; A input; q12 output
function q12 = fcn(z2, z1, p2, p1, gamma_l, rho_l, d_tubo, mu_l, L_tubo, c, A_tubo, g, k_imbocco, k_uscita, A)

k_visc_p = (64*L_tubo) / (rho_l*(d_tubo/mu_l)*(c*A)/A_tubo) * (L_tubo/d_tubo);
caa = (c*A/A_tubo)^2;

AA = -(k_imbocco*caa+k_uscita+1)/(2*g);
BB = -k_visc_p*caa/(2*g);
CC = (z2-z1)+(p2-p1)/gamma_l;

v12 = (-BB - sqrt(BB^2-4*AA*CC)) / (2*AA);

if isnan(v12);
   v12 = 0;
end

q12 = A*c*v12

== matlab function definitivo/Subsystem6/MATLAB Function2 ==
  data: theta input; sezione_piccolo output; r input; h_limite input; h_tappo input
function sezione_piccolo = altezza_sezione_piccolo(theta, r, h_limite, h_tappo)

if h_tappo >= h_limite
    h_tappo = h_limite;     % questa sezione non si apre di più quando si apre il grande
end


m = tan(theta);
y0 = r * m;

xg = r;
yg = y0;

a = sin(pi/2 - theta) * h_tappo;

xr = r - a * sin(theta);
yr = y0+a*cos(theta);


sezione_piccolo = pi * (xg - xr) * a;

== matlab function definitivo/Subsystem6/MATLAB Function3 ==
  data: theta input; sezione_grande output; r input; h_limite input; h_tappo input
function sezione_grande = altezza_sezione_grande(theta, r, h_limite, h_tappo)

if h_tappo < h_limite
    h_tappo = 0;    
else
    h_tappo = h_tappo - h_limite;
end

m = tan(theta);
y0 = r * m;

xg = r;
yg = y0;

a = sin(pi/2 - theta) * h_tappo;

xr = r - a * sin(theta);
yr = y0+a*cos(theta);


sezione_grande = pi * (xg - xr) * a;

== matlab function definitivo/Subsystem7/MATLAB Function2 ==
  data: theta input; sezione_piccolo output; r input; h_limite input; h_tappo input
function sezione_piccolo = altezza_sezione_piccolo(theta, r, h_limite, h_tappo)

if h_tappo >= h_limite
    h_tappo = h_limite;     % questa sezione non si apre di più quando si apre il grande
end


m = tan(theta);
y0 = r * m;

xg = r;
yg = y0;

a = sin(pi/2 - theta) * h_tappo;

xr = r - a * sin(theta);
yr = y0+a*cos(theta);


sezione_piccolo = pi * (xg - xr) * a;

== matlab function definitivo/Subsystem7/MATLAB Function3 ==
  data: theta input; sezione_grande output; r input; h_limite input; h_tappo input
function sezione_grande = altezza_sezione_grande(theta, r, h_limite, h_tappo)

if h_tappo < h_limite
    h_tappo = 0;    
else
    h_tappo = h_tappo - h_limite;
end

m = tan(theta);
y0 = r * m;

xg = r;
yg = y0;

a = sin(pi/2 - theta) * h_tappo;

xr = r - a * sin(theta);
yr = y0+a*cos(theta);


sezione_grande = pi * (xg - xr) * a;

== matlab function definitivo/Subsystem8/MATLAB Function2 ==
  data: z2 input; z1 input; p2 input; p1 input; gamma_l input; rho_l input; d_tubo input; mu_l input; L_tubo input; c input; A_tubo input; g input; k_imbocco input; k_uscita input; A input; q12 output
function q12 = fcn(z2, z1, p2, p1, gamma_l, rho_l, d_tubo, mu_l, L_tubo, c, A_tubo, g, k_imbocco, k_uscita, A)

k_visc_p = (64*L_tubo) / (rho_l*(d_tubo/mu_l)*(c*A)/A_tubo) * (L_tubo/d_tubo);
caa = (c*A/A_tubo)^2;

AA = -(k_imbocco*caa+k_uscita+1)/(2*g);
BB = -k_visc_p*caa/(2*g);
CC = (z2-z1)+(p2-p1)/gamma_l;

v12 = (-BB - sqrt(BB^2-4*AA*CC)) / (2*AA);

if isnan(v12);
   v12 = 0;
end

q12 = A*c*v12

== matlab function definitivo/Subsystem9/MATLAB Function ==
  data: alpha input; h_tappo output; r input; l input; mu input

function h_tappo = manovellismo(alpha, r, l, mu)

h_tappo = (r+l) - (r*cos(alpha) + l/mu*sqrt(mu^2-sin(alpha)^2))

end

== matlab function definitivo/Subsystem10/MATLAB Function ==
  data: alpha input; h_tappo output; r input; l input; mu input

function h_tappo = manovellismo(alpha, r, l, mu)

h_tappo = (r+l) - (r*cos(alpha) + l/mu*sqrt(mu^2-sin(alpha)^2))

end

== matlab function definitivo/Subsystem11/MATLAB Function2 ==
  data: theta input; sezione_piccolo output; r input; h_limite input; h_tappo input
function sezione_piccolo = altezza_sezione_piccolo(theta, r, h_limite, h_tappo)

if h_tappo >= h_limite
    h_tappo = h_limite;     % questa sezione non si apre di più quando si apre il grande
end


m = tan(theta);
y0 = r * m;

xg = r;
yg = y0;

a = sin(pi/2 - theta) * h_tappo;

xr = r - a * sin(theta);
yr = y0+a*cos(theta);


sezione_piccolo = pi * (xg - xr) * a;

== matlab function definitivo/Subsystem11/MATLAB Function3 ==
  data: theta input; sezione_grande output; r input; h_limite input; h_tappo input
function sezione_grande = altezza_sezione_grande(theta, r, h_limite, h_tappo)

if h_tappo < h_limite
    h_tappo = 0;    
else
    h_tappo = h_tappo - h_limite;
end

m = tan(theta);
y0 = r * m;

xg = r;
yg = y0;

a = sin(pi/2 - theta) * h_tappo;

xr = r - a * sin(theta);
yr = y0+a*cos(theta);


sezione_grande = pi * (xg - xr) * a;

== matlab function definitivo/Subsystem12/MATLAB Function2 ==
  data: z2 input; z1 input; p2 input; p1 input; gamma_l input; rho_l input; d_tubo input; mu_l input; L_tubo input; c input; A_tubo input; g input; k_imbocco input; k_uscita input; A input; q12 output
function q12 = fcn(z2, z1, p2, p1, gamma_l, rho_l, d_tubo, mu_l, L_tubo, c, A_tubo, g, k_imbocco, k_uscita, A)

k_visc_p = (64*L_tubo) / (rho_l*(d_tubo/mu_l)*(c*A)/A_tubo) * (L_tubo/d_tubo);
caa = (c*A/A_tubo)^2;

AA = -(k_imbocco*caa+k_uscita+1)/(2*g);
BB = -k_visc_p*caa/(2*g);
CC = (z2-z1)+(p2-p1)/gamma_l;

v12 = (-BB - sqrt(BB^2-4*AA*CC)) / (2*AA);

if isnan(v12);
   v12 = 0;
end

q12 = A*c*v12

== matlab function definitivo/Subsystem14/MATLAB Function2 ==
  data: z2 input; z1 input; p2 input; p1 input; gamma_l input; rho_l input; d_tubo input; mu_l input; L_tubo input; c input; A_tubo input; g input; k_imbocco input; k_uscita input; A input; q12 output
function q12 = fcn(z2, z1, p2, p1, gamma_l, rho_l, d_tubo, mu_l, L_tubo, c, A_tubo, g, k_imbocco, k_uscita, A)

k_visc_p = (64*L_tubo) / (rho_l*(d_tubo/mu_l)*(c*A)/A_tubo) * (L_tubo/d_tubo);
caa = (c*A/A_tubo)^2;

AA = -(k_imbocco*caa+k_uscita+1)/(2*g);
BB = -k_visc_p*caa/(2*g);
CC = (z2-z1)+(p2-p1)/gamma_l;

v12 = (-BB - sqrt(BB^2-4*AA*CC)) / (2*AA);

if isnan(v12);
   v12 = 0;
end

q12 = A*c*v12

== matlab function definitivo/Subsystem3/MATLAB Function2 ==
  data: q11 output; z2 input; z1 input; p2 input; p1 input; gamma_l input; rho_l input; d_tubo input; mu_l input; L_tubo input; c input; A_tubo input; g input; k_imbocco input; k_uscita input; A input; q12 output
function [q11, q12] = fcn(z2, z1, p2, p1, gamma_l, rho_l, d_tubo, mu_l, L_tubo, c, A_tubo, g, k_imbocco, k_uscita, A)

k_visc_p = (64*L_tubo) / (rho_l*(d_tubo/mu_l)*(c*A)/A_tubo) * (L_tubo/d_tubo);
caa = (c*A/A_tubo)^2;

AA = -(k_imbocco*caa+k_uscita+1)/(2*g);
BB = -k_visc_p*caa/(2*g);
CC = (z2-z1)+(p2-p1)/gamma_l;

v11 = (-BB + sqrt(BB^2-4*AA*CC)) / (2*AA); % col - veniva soluzione negativa
v12 = (-BB - sqrt(BB^2-4*AA*CC)) / (2*AA);

if isnan(v11);
   v11 = 0;
end

if isnan(v12);
   v12 = 0;
end


q11 = A*c*v11
q12 = A*c*v12

== matlab function definitivo/Subsystem2/MATLAB Function ==
  data: alpha input; h_tappo output; r input; l input; mu input

function h_tappo = manovellismo(alpha, r, l, mu)

h_tappo = (r+l) - (r*cos(alpha) + l/mu*sqrt(mu^2-sin(alpha)^2))

end

== matlab function definitivo/MATLAB Function2 ==
  data: altezza_liquido input; tau output; L input
function tau = variable_delay(altezza_liquido, L)

    
tau = sqrt(2* (L - ( altezza_liquido) ) / 9.81);

== matlab function definitivo/Subsystem15/MATLAB Function2 ==
  data: theta input; sezione_piccolo output; r input; h_limite input; h_tappo input
function sezione_piccolo = altezza_sezione_piccolo(theta, r, h_limite, h_tappo)

if h_tappo >= h_limite
    h_tappo = h_limite;     % questa sezione non si apre di più quando si apre il grande
end


m = tan(theta);
y0 = r * m;

xg = r;
yg = y0;

a = sin(pi/2 - theta) * h_tappo;

xr = r - a * sin(theta);
yr = y0+a*cos(theta);


sezione_piccolo = pi * (xg - xr) * a;

== matlab function definitivo/Subsystem15/MATLAB Function3 ==
  data: theta input; sezione_grande output; r input; h_limite input; h_tappo input
function sezione_grande = altezza_sezione_grande(theta, r, h_limite, h_tappo)

if h_tappo < h_limite
    h_tappo = 0;    
else
    h_tappo = h_tappo - h_limite;
end

m = tan(theta);
y0 = r * m;

xg = r;
yg = y0;

a = sin(pi/2 - theta) * h_tappo;

xr = r - a * sin(theta);
yr = y0+a*cos(theta);


sezione_grande = pi * (xg - xr) * a;

== matlab function definitivo/Subsystem16/MATLAB Function2 ==
  data: z2 input; z1 input; p2 input; p1 input; gamma_l input; rho_l input; d_tubo input; mu_l input; L_tubo input; c input; A_tubo input; g input; k_imbocco input; k_uscita input; A input; q12 output
function q12 = fcn(z2, z1, p2, p1, gamma_l, rho_l, d_tubo, mu_l, L_tubo, c, A_tubo, g, k_imbocco, k_uscita, A)

k_visc_p = (64*L_tubo) / (rho_l*(d_tubo/mu_l)*(c*A)/A_tubo) * (L_tubo/d_tubo);
caa = (c*A/A_tubo)^2;

AA = -(k_imbocco*caa+k_uscita+1)/(2*g);
BB = -k_visc_p*caa/(2*g);
CC = (z2-z1)+(p2-p1)/gamma_l;

v12 = (-BB - sqrt(BB^2-4*AA*CC)) / (2*AA);

if isnan(v12);
   v12 = 0;
end

q12 = A*c*v12

== matlab function definitivo/Subsystem17/MATLAB Function ==
  data: alpha input; h_tappo output; r input; l input; mu input

function h_tappo = manovellismo(alpha, r, l, mu)

h_tappo = (r+l) - (r*cos(alpha) + l/mu*sqrt(mu^2-sin(alpha)^2))

end

== matlab function definitivo/MATLAB Function3 ==
  data: altezza_liquido input; tau output; L input
function tau = variable_delay(altezza_liquido, L)

    
tau = sqrt(2* (L - ( altezza_liquido) ) / 9.81);

== matlab function definitivo/Subsystem18/MATLAB Function2 ==
  data: theta input; sezione_piccolo output; r input; h_limite input; h_tappo input
function sezione_piccolo = altezza_sezione_piccolo(theta, r, h_limite, h_tappo)

if h_tappo >= h_limite
    h_tappo = h_limite;     % questa sezione non si apre di più quando si apre il grande
end


m = tan(theta);
y0 = r * m;

xg = r;
yg = y0;

a = sin(pi/2 - theta) * h_tappo;

xr = r - a * sin(theta);
yr = y0+a*cos(theta);


sezione_piccolo = pi * (xg - xr) * a;

== matlab function definitivo/Subsystem18/MATLAB Function3 ==
  data: theta input; sezione_grande output; r input; h_limite input; h_tappo input
function sezione_grande = altezza_sezione_grande(theta, r, h_limite, h_tappo)

if h_tappo < h_limite
    h_tappo = 0;    
else
    h_tappo = h_tappo - h_limite;
end

m = tan(theta);
y0 = r * m;

xg = r;
yg = y0;

a = sin(pi/2 - theta) * h_tappo;

xr = r - a * sin(theta);
yr = y0+a*cos(theta);


sezione_grande = pi * (xg - xr) * a;

== matlab function definitivo/Subsystem19/MATLAB Function2 ==
  data: z2 input; z1 input; p2 input; p1 input; gamma_l input; rho_l input; d_tubo input; mu_l input; L_tubo input; c input; A_tubo input; g input; k_imbocco input; k_uscita input; A input; q12 output
function q12 = fcn(z2, z1, p2, p1, gamma_l, rho_l, d_tubo, mu_l, L_tubo, c, A_tubo, g, k_imbocco, k_uscita, A)

k_visc_p = (64*L_tubo) / (rho_l*(d_tubo/mu_l)*(c*A)/A_tubo) * (L_tubo/d_tubo);
caa = (c*A/A_tubo)^2;

AA = -(k_imbocco*caa+k_uscita+1)/(2*g);
BB = -k_visc_p*caa/(2*g);
CC = (z2-z1)+(p2-p1)/gamma_l;

v12 = (-BB - sqrt(BB^2-4*AA*CC)) / (2*AA);

if isnan(v12);
   v12 = 0;
end

q12 = A*c*v12

== matlab function definitivo/Subsystem20/MATLAB Function ==
  data: alpha input; h_tappo output; r input; l input; mu input

function h_tappo = manovellismo(alpha, r, l, mu)

h_tappo = (r+l) - (r*cos(alpha) + l/mu*sqrt(mu^2-sin(alpha)^2))

end

== matlab function definitivo/Subsystem1/MATLAB Function ==
  data: alpha input; h_tappo output; r input; l input; mu input

function h_tappo = manovellismo(alpha, r, l, mu)

h_tappo = (r+l) - (r*cos(alpha) + l/mu*sqrt(mu^2-sin(alpha)^2))

end

== matlab function definitivo/MATLAB Function1 ==
  data: altezza_liquido input; tau output; L input
function tau = variable_delay(altezza_liquido, L)

    
tau = sqrt(2* (L - ( altezza_liquido) ) / 9.81);

== matlab function definitivo/Subsystem13/MATLAB Function2 ==
  data: theta input; sezione_piccolo output; r input; h_limite input; h_tappo input
function sezione_piccolo = altezza_sezione_piccolo(theta, r, h_limite, h_tappo)

if h_tappo >= h_limite
    h_tappo = h_limite;     % questa sezione non si apre di più quando si apre il grande
end


m = tan(theta);
y0 = r * m;

xg = r;
yg = y0;

a = sin(pi/2 - theta) * h_tappo;

xr = r - a * sin(theta);
yr = y0+a*cos(theta);


sezione_piccolo = pi * (xg - xr) * a;

== matlab function definitivo/Subsystem13/MATLAB Function3 ==
  data: theta input; sezione_grande output; r input; h_limite input; h_tappo input
function sezione_grande = altezza_sezione_grande(theta, r, h_limite, h_tappo)

if h_tappo < h_limite
    h_tappo = 0;    
else
    h_tappo = h_tappo - h_limite;
end

m = tan(theta);
y0 = r * m;

xg = r;
yg = y0;

a = sin(pi/2 - theta) * h_tappo;

xr = r - a * sin(theta);
yr = y0+a*cos(theta);


sezione_grande = pi * (xg - xr) * a;

== matlab function definitivo/Subsystem4/MATLAB Function2 ==
  data: z2 input; z1 input; p2 input; p1 input; gamma_l input; rho_l input; d_tubo input; mu_l input; L_tubo input; c input; A_tubo input; g input; k_imbocco input; k_uscita input; A input; q12 output
function q12 = fcn(z2, z1, p2, p1, gamma_l, rho_l, d_tubo, mu_l, L_tubo, c, A_tubo, g, k_imbocco, k_uscita, A)

k_visc_p = (64*L_tubo) / (rho_l*(d_tubo/mu_l)*(c*A)/A_tubo) * (L_tubo/d_tubo);
caa = (c*A/A_tubo)^2;

AA = -(k_imbocco*caa+k_uscita+1)/(2*g);
BB = -k_visc_p*caa/(2*g);
CC = (z2-z1)+(p2-p1)/gamma_l;

v12 = (-BB - sqrt(BB^2-4*AA*CC)) / (2*AA);

if isnan(v12);
   v12 = 0;
end

q12 = A*c*v12
